simulink model "HDLRemoveToneMapping"  (R2024a)
settings: Solver=FixedStepDiscrete  StartTime=0.0  StopTime=stopTime  RelTol=1e-3
undefined symbols (not defined in the file): CONST, psduSize
libraries: dspsrcs4 x3, whdlutilities x1, HDL_ieee_8021513 x1
settings Model: DataTypeOverride=Off  Creator=cotti  LastModifiedBy=cotti
settings OptimizationCC: BlockReduction=off  ConditionallyExecuteInputs=off  DefaultParameterBehavior=Inlined  InheritOutputTypeSmallerThanSingle=on
settings DebuggingCC: ArtificialAlgebraicLoopMsg=error  SingleTaskRateTransMsg=error
settings HardwareCC: ProdBitPerPointer=32  ProdBitPerSizeT=32  ProdBitPerPtrDiffT=32  ProdLargestAtomicFloat=None  ProdIntDivRoundTo=Undefined  ProdEndianess=Unspecified  ProdWordSize=32  ProdHWDeviceType=ASIC/FPGA->ASIC/FPGA  TargetBitPerLong=64  TargetBitPerPointer=64  TargetBitPerSizeT=64  TargetBitPerPtrDiffT=64  TargetLongLongMode=on  TargetIntDivRoundTo=Zero  TargetEndianess=LittleEndian  TargetWordSize=64  TargetHWDeviceType=Custom Processor->MATLAB Host Computer  ProdEqTarget=off

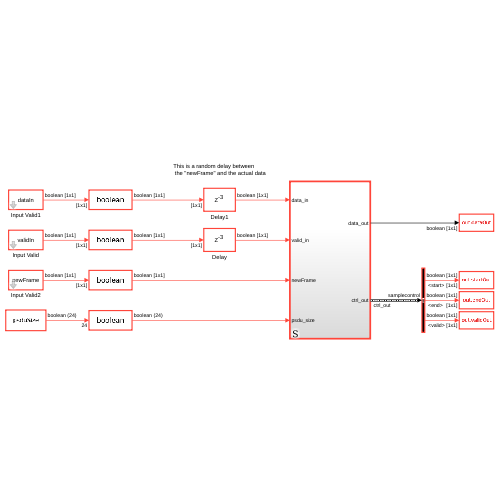
[thumbnail: Simulink's stored preview of the top-level diagram]
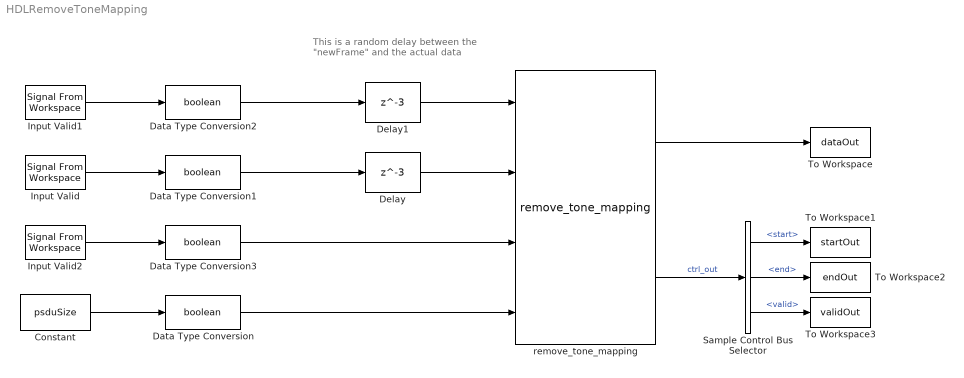
== system HDLRemoveToneMapping ==
  note: This is a random delay between
      |  the "newFrame" and the actual data
  Constant : Constant  Value=psduSize  SampleTime=1/CONST.fs
  Data Type Conversion{,1..3} (4 alike) : DataTypeConversion  OutDataTypeStr=boolean  SaturateOnIntegerOverflow=off  RndMeth=Floor
  Delay : Delay  DelayLength=3  InitialCondition=0  UseCircularBuffer=on
  Delay1 : Delay  DelayLength=3  InitialCondition=0  UseCircularBuffer=on
  Input Valid : dspsrcs4/Signal From Workspace  X=validIn  Ts=1/CONST.fs  nsamps=1  OutputAfterFinalValue=Setting to zero  ignoreOrWarnInputAndFrameLengths=off  OutputFrames=off
  Input Valid1 : dspsrcs4/Signal From Workspace  X=dataIn  Ts=1/CONST.fs  nsamps=1  OutputAfterFinalValue=Setting to zero  ignoreOrWarnInputAndFrameLengths=off  OutputFrames=off
  Input Valid2 : dspsrcs4/Signal From Workspace  X=newFrame  Ts=1/CONST.fs  nsamps=1  OutputAfterFinalValue=Setting to zero  ignoreOrWarnInputAndFrameLengths=off  OutputFrames=off
  Sample Control Bus Selector : whdlutilities/Sample Control Bus Selector  OutputSignals=start,end,valid
  To Workspace : ToWorkspace  VariableName=dataOut  SampleTime=1/CONST.fs
      settings: Save2DSignal=2-D array (concatenate along first dimension)
  To Workspace1 : ToWorkspace  VariableName=startOut  SampleTime=1/CONST.fs
      settings: Save2DSignal=2-D array (concatenate along first dimension)
  To Workspace2 : ToWorkspace  VariableName=endOut  SampleTime=1/CONST.fs
      settings: Save2DSignal=2-D array (concatenate along first dimension)
  To Workspace3 : ToWorkspace  VariableName=validOut  SampleTime=1/CONST.fs
      settings: Save2DSignal=2-D array (concatenate along first dimension)
  remove_tone_mapping : HDL_ieee_8021513/remove_tone_mapping  SystemSampleTime=-1  VariantActivationTime=update diagram  AllowFlexibleInterface=on  Latency=0  AutoFrameSizeCalculation=off
      settings: SourceProductName=HDL IEEE 8021513
  wires:
  Constant/1 -> Data Type Conversion/1
  Input Valid/1 -> Data Type Conversion1/1
  Data Type Conversion1/1 -> Delay/1
  Input Valid1/1 -> Data Type Conversion2/1
  Data Type Conversion2/1 -> Delay1/1
  Sample Control Bus Selector/2 -> To Workspace2/1  "<end>"
  Sample Control Bus Selector/3 -> To Workspace3/1  "<valid>"
  Sample Control Bus Selector/1 -> To Workspace1/1  "<start>"
  remove_tone_mapping/2 -> Sample Control Bus Selector/1  "ctrl_out"
  remove_tone_mapping/1 -> To Workspace/1
  Data Type Conversion/1 -> remove_tone_mapping/4
  Data Type Conversion3/1 -> remove_tone_mapping/3
  Input Valid2/1 -> Data Type Conversion3/1
  Delay/1 -> remove_tone_mapping/2
  Delay1/1 -> remove_tone_mapping/1
